simulink model "controller"  (R2023b)
settings: Solver=FixedStepAuto  StartTime=0.0  StopTime=10.0  FixedStep=1/10  RelTol=1e-3  EnableMultiTasking=on
libraries: simulink x1
settings Model: ExtModeTrigDuration=2  Creator=DAUIN-Win10  LastModifiedBy=dadog
settings OptimizationCC: EnhancedBackFolding=on  PassReuseOutputArgsAs=Individual arguments  ZeroExternalMemoryAtStartup=off  ZeroInternalMemoryAtStartup=off  MaxStackSize=64  OptimizeBlockOrder=speed  DifferentSizesBufferReuse=on  OptimizationCustomize=off  EfficientTunableParamExpr=on
settings DebuggingCC: ParameterTunabilityLossMsg=error  UnconnectedInputMsg=warning  UnconnectedOutputMsg=warning  UnconnectedLineMsg=warning
settings HardwareCC: ProdBitPerInt=16  ProdBitPerPointer=16  ProdBitPerSizeT=16  ProdBitPerPtrDiffT=16  ProdLargestAtomicFloat=None  ProdWordSize=8  ProdHWDeviceType=Atmel->AVR
settings ModelReferenceCC: EnableRefExpFcnMdlSchedulingChecks=on
settings SFSimCC: MATLABDynamicMemAlloc=off
settings RTWCC: Description=Embedded Coder  SystemTargetFile=ert.tlc  HardwareBoard=Arduino Uno  TemplateMakefile=ert_default_tmf  Toolchain=Arduino AVR  BuildConfiguration=Faster Runs  DLArmComputeVersion=19.05
settings CodeAppCC: ForceParamTrailComments=on  IgnoreCustomStorageClasses=off  OperatorAnnotations=on  SimulinkDataObjDesc=on  SFDataObjDesc=on  InsertBlockDesc=on
settings ERTTargetCC: SupportContinuousTime=on  SupportVariableSizeSignals=on  ExtModeTransport=3  ExtModeStaticAlloc=on  ExtModeStaticAllocSize=250  ExtModeMexFile=ext_xcp  ExtModeIntrfLevel=Level2 - Open

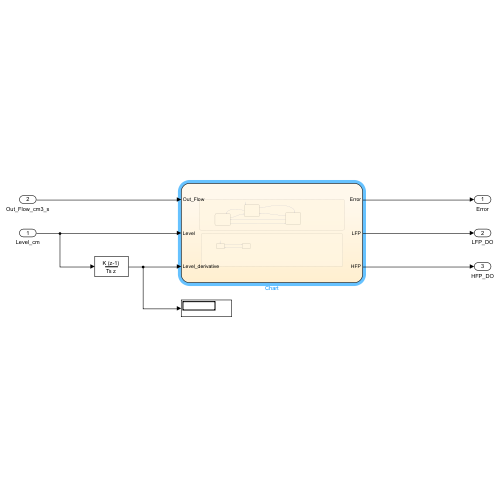
[thumbnail: Simulink's stored preview of the top-level diagram]
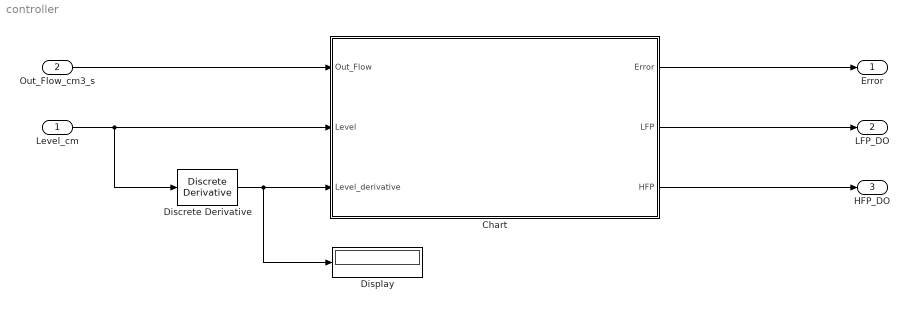
== system controller ==
  Level_cm : Inport
  Out_Flow_cm3_s : Inport  Port=2
  Chart : Stateflow chart  TreatAsAtomicUnit=on
  Discrete Derivative : simulink/Discrete/Discrete Derivative  gainval=1.0  ICPrevScaledInput=0.0  OutMin=[]  OutMax=[]  OutDataType=fixdt(1, 16)  OutScaling=2^-10  DoSatur=off
  Display : Display
  Error : Outport  OutDataTypeStr=uint8
  LFP_DO : Outport  Port=2  OutDataTypeStr=boolean
  HFP_DO : Outport  Port=3  OutDataTypeStr=boolean
  wires:
  Level_cm/1 -> Discrete Derivative/1, Chart/2(Level)
  Out_Flow_cm3_s/1 -> Chart/1(Out_Flow)
  Chart/1(Error) -> Error/1
  Chart/2(LFP) -> LFP_DO/1
  Chart/3(HFP) -> HFP_DO/1
  Discrete Derivative/1 -> Display/1, Chart/3(Level_derivative)

== stateflow chart controller/Chart ==
  state Controller [parallel]
    settings: executionOrder=1
    state OFF
      en:
      HFP=false;
      LFP=false;
    state LFP_ON
      du:
      HFP=false;
      LFP=true;
    state HFP_ON
      du:
      HFP=true;
      LFP=false;
    (default) -> OFF
    OFF -> LFP_ON [order 2] : [Level_derivative<0 && Level < 175]
    OFF -> HFP_ON [order 1] : [Level_derivative<0 && Level < 150]
    LFP_ON -> OFF [order 1] : [Level_derivative>0 && Level > 180]
    HFP_ON -> OFF [order 2] : [Level > 180]
    LFP_ON -> HFP_ON [order 2] : [Level_derivative<0 && Level < 150 && Error != 2 || Error == 1]
    HFP_ON -> LFP_ON [order 1] : [Level_derivative>0 && Level > 155 || Error == 2]
  state Monitor [parallel]
    settings: executionOrder=2
    state No_ERR
      en:
      Error = 0;
    state ERR
      en:
      Error = 1;
    (default) -> No_ERR
    No_ERR -> ERR : [Level < 130 || Level > 190]
    ERR -> No_ERR : [Level >= 130 && Level <= 190]
  data: Out_Flow input double size=1; Level input double; Error output uint8 size=1; LFP output boolean; HFP output boolean; Level_derivative input double
